simulink model "Mechanical_Motor_Models_TESTING"  (R2019b)
settings: Solver=VariableStepAuto  StartTime=0.0  StopTime=10.0  FixedStep=0.0001  RelTol=1e-3
undefined symbols (not defined in the file): EB, EJ, EKb, EKm, EL, ENominal_V, ER, GB, GJ, GKb, GKm, GL, GNominal_V, GR, SB, SJ, SKb, SKm, SL, SR, WB, WJ, WKb, WKm, WL, WNominal_V
libraries: cstblocks x4
settings Model: Creator=harsh  LastModifiedBy=harsh

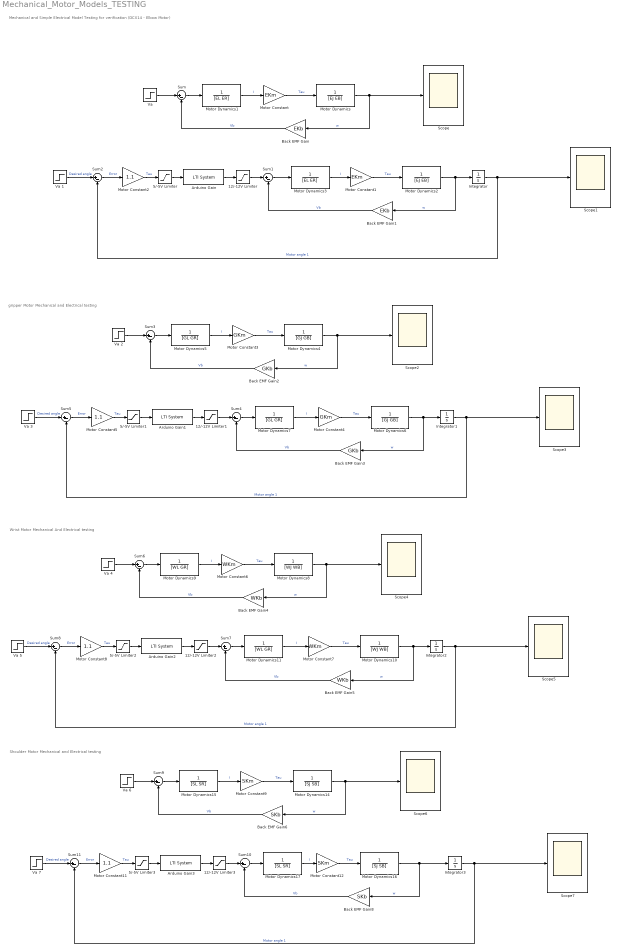
== system Mechanical_Motor_Models_TESTING ==
  note: Shoulder Motor Mechanical and Electrical testing
  note: Wrist Motor Mechanical And Electrical testing
  note: gripper Motor Mechanical and Electrical testing
  note: Mechanical and Simple Electrical Model Testing for verification (DCX14 - Elbow Motor)
  12/-12V Limiter{,1..3} (4 alike) : Saturate  UpperLimit=12  LowerLimit=-12
  5/-5V Limiter{,1..3} (4 alike) : Saturate  UpperLimit=5  LowerLimit=-5
  Arduino Gain{,1..3} (4 alike) : cstblocks/LTI System  sys=OPAMP  IC=[]
  Back EMF Gain : Gain  Gain=EKb
  Back EMF Gain1 : Gain  Gain=EKb
  Back EMF Gain2 : Gain  Gain=GKb
  Back EMF Gain3 : Gain  Gain=GKb
  Back EMF Gain4 : Gain  Gain=WKb
  Back EMF Gain5 : Gain  Gain=WKb
  Back EMF Gain6 : Gain  Gain=SKb
  Back EMF Gain8 : Gain  Gain=SKb
  Integrator{,1..3} (4 alike) : Integrator
  Motor Constant : Gain  Gain=EKm
  Motor Constant1 : Gain  Gain=EKm
  Motor Constant{2,5,8,11} (4 alike) : Gain  Gain=1.1
  Motor Constant12 : Gain  Gain=SKm
  Motor Constant3 : Gain  Gain=GKm
  Motor Constant4 : Gain  Gain=GKm
  Motor Constant6 : Gain  Gain=WKm
  Motor Constant7 : Gain  Gain=WKm
  Motor Constant9 : Gain  Gain=SKm
  Motor Dynamics : TransferFcn  Denominator=[EJ EB]
  Motor Dynamics1 : TransferFcn  Denominator=[EL ER]
  Motor Dynamics10 : TransferFcn  Denominator=[WJ WB]
  Motor Dynamics11 : TransferFcn  Denominator=[WL GR]
  Motor Dynamics14 : TransferFcn  Denominator=[SJ SB]
  Motor Dynamics15 : TransferFcn  Denominator=[SL SR]
  Motor Dynamics16 : TransferFcn  Denominator=[SJ SB]
  Motor Dynamics17 : TransferFcn  Denominator=[SL SR]
  Motor Dynamics2 : TransferFcn  Denominator=[EJ EB]
  Motor Dynamics3 : TransferFcn  Denominator=[EL ER]
  Motor Dynamics4 : TransferFcn  Denominator=[GJ GB]
  Motor Dynamics5 : TransferFcn  Denominator=[GL GR]
  Motor Dynamics6 : TransferFcn  Denominator=[GJ GB]
  Motor Dynamics7 : TransferFcn  Denominator=[GL GR]
  Motor Dynamics8 : TransferFcn  Denominator=[WJ WB]
  Motor Dynamics9 : TransferFcn  Denominator=[WL GR]
  Scope{,1..7} (8 alike) : Scope
  Sum{,1..11} (12 alike) : Sum  Inputs=|+-
  "Va " : Step  After=ENominal_V  SampleTime=0
  Va {1,3,5,7} (4 alike) : Step  After=pi/2  SampleTime=0
  Va 2 : Step  After=GNominal_V  SampleTime=0
  Va 4 : Step  After=WNominal_V  SampleTime=0
  Va 6 : Step  After=WNominal_V  SampleTime=0
  wires:
  Back EMF Gain/1 -> Sum/2  "Vb"
  Motor Dynamics/1 -> Scope/1, Back EMF Gain/1  "w"
  Motor Dynamics1/1 -> Motor Constant/1  "I"
  Motor Constant/1 -> Motor Dynamics/1  "Tau"
  Sum/1 -> Motor Dynamics1/1
  "Va "/1 -> Sum/1
  Va 1/1 -> Sum2/1  "Desired angle"
  Sum2/1 -> Motor Constant2/1  "Error"
  Arduino Gain/1 -> 12/-12V Limiter/1
  5/-5V Limiter/1 -> Arduino Gain/1
  Back EMF Gain1/1 -> Sum1/2  "Vb"
  Motor Dynamics3/1 -> Motor Constant1/1  "I"
  Sum1/1 -> Motor Dynamics3/1
  Motor Constant1/1 -> Motor Dynamics2/1  "Tau"
  Motor Dynamics2/1 -> Back EMF Gain1/1, Integrator/1  "w"
  12/-12V Limiter/1 -> Sum1/1
  Integrator/1 -> Scope1/1, Sum2/2  "Motor angle 1"
  Motor Constant2/1 -> 5/-5V Limiter/1  "Tau"
  Motor Dynamics6/1 -> Back EMF Gain3/1, Integrator1/1  "w"
  Motor Constant5/1 -> 5/-5V Limiter1/1  "Tau"
  5/-5V Limiter1/1 -> Arduino Gain1/1
  Back EMF Gain3/1 -> Sum4/2  "Vb"
  12/-12V Limiter1/1 -> Sum4/1
  Arduino Gain1/1 -> 12/-12V Limiter1/1
  Back EMF Gain2/1 -> Sum3/2  "Vb"
  Va 3/1 -> Sum5/1  "Desired angle"
  Motor Dynamics7/1 -> Motor Constant4/1  "I"
  Sum4/1 -> Motor Dynamics7/1
  Va 2/1 -> Sum3/1
  Motor Dynamics5/1 -> Motor Constant3/1  "I"
  Sum3/1 -> Motor Dynamics5/1
  Motor Constant3/1 -> Motor Dynamics4/1  "Tau"
  Sum5/1 -> Motor Constant5/1  "Error"
  Motor Constant4/1 -> Motor Dynamics6/1  "Tau"
  Motor Dynamics4/1 -> Scope2/1, Back EMF Gain2/1  "w"
  Integrator1/1 -> Scope3/1, Sum5/2  "Motor angle 1"
  Motor Constant7/1 -> Motor Dynamics10/1  "Tau"
  Motor Dynamics11/1 -> Motor Constant7/1  "I"
  Motor Constant8/1 -> 5/-5V Limiter2/1  "Tau"
  Motor Dynamics9/1 -> Motor Constant6/1  "I"
  Sum8/1 -> Motor Constant8/1  "Error"
  Va 4/1 -> Sum6/1
  Motor Constant6/1 -> Motor Dynamics8/1  "Tau"
  Sum6/1 -> Motor Dynamics9/1
  Back EMF Gain5/1 -> Sum7/2  "Vb"
  Va 5/1 -> Sum8/1  "Desired angle"
  Motor Dynamics8/1 -> Scope4/1, Back EMF Gain4/1  "w"
  5/-5V Limiter2/1 -> Arduino Gain2/1
  Integrator2/1 -> Scope5/1, Sum8/2  "Motor angle 1"
  Back EMF Gain4/1 -> Sum6/2  "Vb"
  Motor Dynamics10/1 -> Back EMF Gain5/1, Integrator2/1  "w"
  Arduino Gain2/1 -> 12/-12V Limiter2/1
  Sum7/1 -> Motor Dynamics11/1
  12/-12V Limiter2/1 -> Sum7/1
  Va 7/1 -> Sum11/1  "Desired angle"
  Sum9/1 -> Motor Dynamics15/1
  Motor Constant9/1 -> Motor Dynamics14/1  "Tau"
  Motor Dynamics15/1 -> Motor Constant9/1  "I"
  Motor Constant11/1 -> 5/-5V Limiter3/1  "Tau"
  12/-12V Limiter3/1 -> Sum10/1
  Back EMF Gain6/1 -> Sum9/2  "Vb"
  Motor Dynamics14/1 -> Scope6/1, Back EMF Gain6/1  "w"
  Arduino Gain3/1 -> 12/-12V Limiter3/1
  Integrator3/1 -> Scope7/1, Sum11/2  "Motor angle 1"
  Sum11/1 -> Motor Constant11/1  "Error"
  5/-5V Limiter3/1 -> Arduino Gain3/1
  Va 6/1 -> Sum9/1
  Back EMF Gain8/1 -> Sum10/2  "Vb"
  Sum10/1 -> Motor Dynamics17/1
  Motor Dynamics17/1 -> Motor Constant12/1  "I"
  Motor Constant12/1 -> Motor Dynamics16/1  "Tau"
  Motor Dynamics16/1 -> Back EMF Gain8/1, Integrator3/1  "w"
